simulink model "lab_3_simulink"  (R2020b)
settings: Solver=VariableStepAuto  StartTime=0.0  StopTime=10.0  RelTol=1e-3
InitFcn:
  | tau = 0.01
values from neighbouring files (symbols this model uses):
  k_1 = 2.0    (= 2)    [lab_3.m]
  k_4 = 1.0    (= 1)    [lab_3.m]
  T_2 = 3.0    (= 3)    [lab_3.m]
  T_31 = 1.5    [lab_3.m]
  T_32 = 1.0    (= 1)    [lab_3.m]
  tau_2 = 4.0    (= 4)    [lab_3.m]
  zeta_31 = 0.25    [lab_3.m]
  zeta_32 = 0.10    (= 0.1)    [lab_3.m]
settings Model: Creator=trene  LastModifiedBy=trene

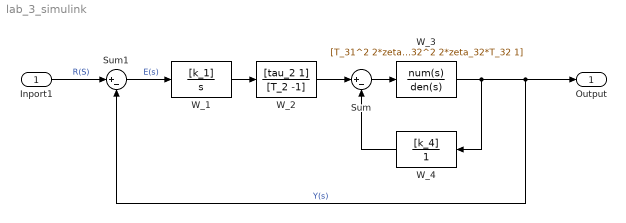
== system lab_3_simulink ==
  Inport1 : Inport
  Sum : Sum  Inputs=|+-
  Sum1 : Sum  Inputs=|+-
  W_1 : TransferFcn  Numerator=[k_1]  Denominator=[1 0]
  W_2 : TransferFcn  Numerator=[tau_2 1]  Denominator=[T_2 -1]
  W_3 : TransferFcn  Numerator=[T_31^2 2*zeta_31*T_31 1]  Denominator=[T_32^2 2*zeta_32*T_32 1]
  W_4 : TransferFcn  Numerator=[k_4]  Denominator=[1]
  Output : Outport
  wires:
  W_3/1 -> Sum1/2, Output/1, W_4/1  "Y(s)"
  Sum/1 -> W_3/1
  W_2/1 -> Sum/1
  W_4/1 -> Sum/2
  W_1/1 -> W_2/1
  Sum1/1 -> W_1/1  "E(s)"
  Inport1/1 -> Sum1/1  "R(S)"
